simulink model "mpc_v1"  (R2020b)
settings: Solver=FixedStepAuto  StartTime=0.0  StopTime=t_sim  FixedStep=Ts  RelTol=1e-3
values from neighbouring files (symbols this model uses):
  A_bar = zeros(n*(Np+1), n)    [main.m]
  B_bar = zeros(n*(Np+1), q*Np)    [main.m]
  C = [1 0 0 0; 0 1 0 0]    [main.m]
  C_bar = zeros(p*(Np+1), n)    [main.m]
  D_bar = zeros(p*(Np+1), q*Np)    [main.m]
  dU_bound = ones(q*Np, 1)*du_bound    [main.m]
  Np = 50    [main.m]
  q = size(B,2)    [main.m]
  Q_bar = blkdiag(Q_cell{:})    [main.m]
  R_bar = blkdiag(R_cell{:})    [main.m]
  ref = [target]    [main.m]
  Ts = 0.1    [main.m]
  U0 = zeros(q*Np, 1)    [main.m]
  U_bound = ones(q*Np, 1)*u_bound    [main.m]
  x0 = [2; 1; 0; 0]    [main.m]
  X_bound = ones(n*(Np+1), 1)*x_bound    [main.m]
undefined symbols (not defined in the file or in its folder): Ad, Bd
settings Model: Creator=vince  LastModifiedBy=vince
settings DataIOCC: ReturnWorkspaceOutputs=off

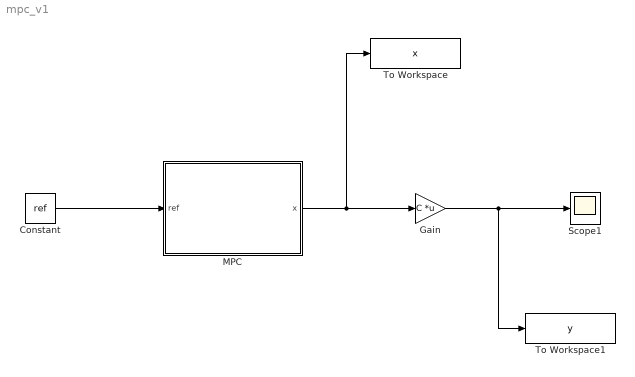
== system mpc_v1 ==
  Constant : Constant  Value=ref  SampleTime=Ts
  Gain : Gain  Gain=C  Multiplication=Matrix(K*u) (u vector)
  MPC : Subsystem
  Scope1 : Scope
  To Workspace : ToWorkspace  VariableName=x  SaveFormat=Timeseries  SampleTime=-1
  To Workspace1 : ToWorkspace  VariableName=y  SaveFormat=Timeseries  SampleTime=-1
  wires:
  Constant/1 -> MPC/1(ref)
  Gain/1 -> Scope1/1, To Workspace1/1
  MPC/1(x) -> Gain/1, To Workspace/1

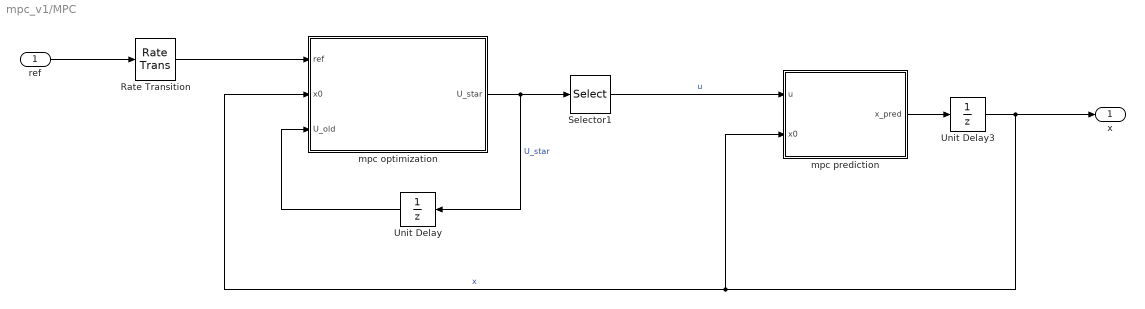
== system mpc_v1/MPC ==
  ref : Inport
  Rate Transition : RateTransition  OutPortSampleTime=Ts
  Selector1 : Selector  InputPortWidth=q*Np  IndexOptions=Index vector (dialog)  Indices=1:q  OutputSizes=1
  Unit Delay : UnitDelay  InitialCondition=U0  SampleTime=Ts  HasFrameUpgradeWarning=on
  Unit Delay3 : UnitDelay  InitialCondition=x0  SampleTime=Ts  HasFrameUpgradeWarning=on
  mpc optimization : MATLAB Function  TreatAsAtomicUnit=on
  mpc prediction : MATLAB Function  TreatAsAtomicUnit=on
  x : Outport
  wires:
  mpc prediction/1(x_pred) -> Unit Delay3/1
  mpc optimization/1(U_star) -> Selector1/1, Unit Delay/1  "U_star"
  Selector1/1 -> mpc prediction/1(u)  "u"
  Rate Transition/1 -> mpc optimization/1(ref)
  Unit Delay3/1 -> mpc optimization/2(x0), mpc prediction/2(x0), x/1  "x"
  Unit Delay/1 -> mpc optimization/3(U_old)
  ref/1 -> Rate Transition/1

== matlab function mpc_v1/MPC/mpc optimization ==
  data: ref input; U_star output; x0 input; U_old input; q parameter; Np parameter; A_bar parameter; B_bar parameter; C_bar parameter; D_bar parameter; R_bar parameter; Q_bar parameter; X_bound parameter; U_bound parameter; dU_bound parameter
function U_star  = mpc_optimization(ref, x0, U_old, q, Np, A_bar, B_bar, C_bar, D_bar, R_bar, Q_bar, X_bound, U_bound, dU_bound)
%% Documentation
%{
    INCOME: ref, x, U_old
    OUTCOME: U*
%}



%% Constraints

REF = repmat(ref, Np+1, 1);

X_min = X_bound(:,1);
X_max = X_bound(:,2);
U_min = U_bound(:,1);
U_max = U_bound(:,2);
dU_min = dU_bound(:,1);
dU_max = dU_bound(:,2);


A_ineq = [-B_bar; B_bar;
        -eye(q*Np); eye(q*Np); 
        -eye(q*Np); eye(q*Np)];
b_ineq = [-X_min+A_bar*x0; X_max-A_bar*x0;
        -U_min; U_max;
        -dU_min-U_old; dU_max+U_old];


    
%% Objective function

H = R_bar + D_bar'*Q_bar*D_bar;
H = (H+H')/2;
f = (C_bar*x0-REF)'*Q_bar*(D_bar);



%% Optimization: J(u(k)) = U(k)'*H*U(k) + f'*U(k)

coder.extrinsic('quadprog');
% options = optimoptions('quadprog', 'Algorithm', 'active-set', 'Display', 'iter');

U_star = zeros(q*Np, 1);
U_star = quadprog(H, f, A_ineq, b_ineq, [], [], [], [], []);

== matlab function mpc_v1/MPC/mpc prediction ==
  data: u input; x_pred output; x0 input; Ad parameter; Bd parameter
function x_pred = mpc_prediction(u, x0, Ad, Bd)

x = x0;
x_pred = Ad*x + Bd*u;
